simulink model "ECE411_ProjectTemplateSim2"  (R2021b)
settings: Solver=FixedStepDiscrete  StartTime=0.0  StopTime=10  FixedStep=Ts  RelTol=1e-3  EnableMultiTasking=on
PreLoadFcn:
  | ee_bldc_speed_control_data;
StopFcn:
  | ee_addSimlogTimeStamp(bdroot)
values from neighbouring files (symbols this model uses):
  Bm = 42e-3    (= 0.042)    [Wooter_parameters.m]
  Drive_Idc_limit = 200    [Wooter_parameters.m]
  eff_radius = r_wheel/G_ratio    (= 0.034375)    [Wooter_parameters.m]
  I_cmd_manual_step = 133    [Wooter_parameters.m]
  Ki_Idc_Regulator = 5.723    [Wooter_parameters.m]
  Ki_vel_Regulator = 5    [Wooter_parameters.m]
  Kp_Idc_Regulator = 0.286    [Wooter_parameters.m]
  Kp_vel_Regulator = 5    [Wooter_parameters.m]
  p = 4    [Wooter_parameters.m]
  RPM_max = 4259    [Wooter_parameters.m]
  tau_Te_filter = 1/(2*pi*10)    (= 0.0159154943092)    [Wooter_parameters.m]
  Tsc = 1e-4    (= 0.0001)    [Wooter_parameters.m]
  Vdc_max = 72    [Wooter_parameters.m]
  vel_0 = 0    [Wooter_parameters.m]
  vel_1 = 11.11    [Wooter_parameters.m]
  vel_2 = 13.889    [Wooter_parameters.m]
  vel_3 = 9.722    [Wooter_parameters.m]
libraries: nesl_utility x16, fl_lib x10, ee_lib x8, eeDiscretePi x2, eeGeneralControl x1
CloseFcn:
  | try,close(h1_ee_bldc_speed_control),end
  | clear h1_ee_bldc_speed_control
  | 
  | clear simlog_ee_bldc_speed_control
  | clear logsout_ee_bldc_speed_control
Description:
  | BLDC Speed Control
settings Model: Creator=The MathWorks, Inc.  LastModifiedBy=divad
settings SolverCC: AlgebraicLoopSolver=TrustRegion
settings DataIOCC: MaxDataPoints=210000  ReturnWorkspaceOutputs=off  SignalLoggingName=logsout_ee_bldc_speed_control
settings OptimizationCC: LifeSpan=inf
settings DebuggingCC: UnderspecifiedInitializationDetection=Classic  MergeDetectMultiDrivingBlocksExec=none  SFUnexpectedBacktrackingDiag=warning  SFNoUnconditionalDefaultTransitionDiag=warning  SFExecutionAtInitializationDiag=none  SFMachineParentedDataDiag=warning  ArithmeticOperatorsInVariantConditions=warning
settings SFSimCC: SimUseLocalCustomCode=off  CustomCodeUndefinedFunction=UseInterfaceOnly
settings RTWCC: RTWUseLocalCustomCode=off
settings CodeAppCC: StateflowObjectComments=on
settings GRTTargetCC: TargetLangStandard=C89/C90 (ANSI)
settings ConfigComp: CovMetricSettings=dw  CovSaveCumulativeToWorkspaceVar=on  CovSaveSingleToWorkspaceVar=on  CovExternalEMLEnable=off
settings SimscapeCC: SimscapeNormalizeSystem=off  SimscapeLogType=all  SimscapeLogSimulationStatistics=on  SimscapeLogName=simlog_ee_bldc_speed_control  SimscapeLogDataHistory=210000

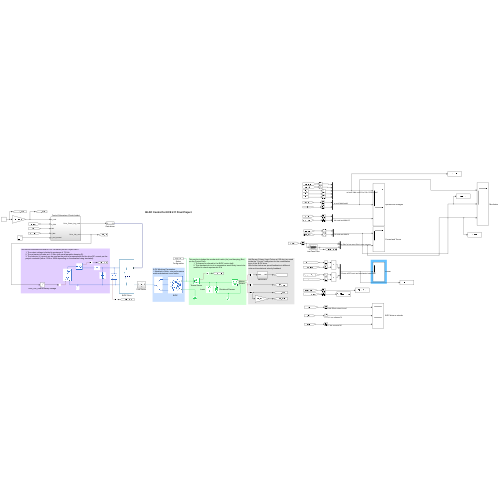
[thumbnail: Simulink's stored preview of the top-level diagram]
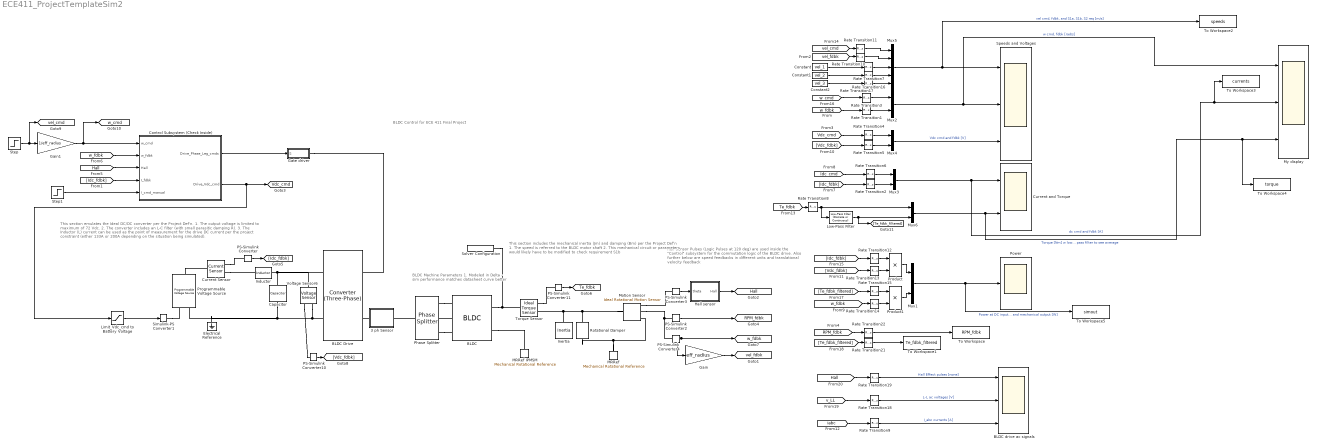
== system ECE411_ProjectTemplateSim2 ==
  note: Hall Sensor Pulses (Logic Pulses at 120 deg) are used inside the "Control" subsystem for the commutation logic of the BLDC drive.
      | Also further below are speed feedbacks in different units and translational velocity feedback
  note: This section emulates the Ideal DC/DC converter per the Project Def'n.
      | 1. The output voltage is limited to maximum of 72 Vdc.
      | 2. The converter includes an L-C filter (with small parasitic damping R).
      | 3. The Inductor (L) current can be used as the point of measurement for the drive DC current per the project constraint (either 133A or 200A depending on the situation being simulated).
  note: BLDC Control for ECE 411 Final Project
  note: This section includes the mechanical inertia (Jm) and damping (Bm) per the Project Def'n
      | 1. The speed is referred to the BLDC motor shaft
      | 2. This mechanical circuit or parameters would likely have to be modified to check requirement S1b
  note: BLDC Machine Parameters
      | 1. Modeled in Delta - sim performance matches datasheet curve better
  3 ph Sensor : Subsystem
  BLDC : ee_lib/Electromechanical/Permanent Magnet/BLDC  port_option=ee.enum.threePhasePort.expanded  winding_type=ee.enum.statorconnection.delta  rotor_param=ee.enum.pmsm.backemf.trapezoidbackemf  pm_flux_linkage=0.175 N*m/A  theta_constant=pi / (2*p) rad  emf_max=Vdc_max V  w_meas=RPM_max rpm  DphiDtheta_tab=[0, -.1528, -.1528, .1528, .1528, 0] Wb/rad  back_emf_tab=[0, -9.6, -9.6, 9.6, 9.6, 0] V  rotor_angle_tab=[0, 7.5, 22.5, 37.5, 52.5, 60] deg  nPolePairs=p  axes_param=ee.enum.rotorangle.qaxis  stator_param=ee.enum.statorparam.LsLmMs  machine_param=ee.enum.dqparameterization.constant  Ld=0.00022 H  Lq=0.00022 H  idVec=[-200, 0, 200] A  iqVec=[-200, 0, 200] A  LdMatrix=0.00022 * ones(3, 3) H  LqMatrix=0.00022 * ones(3, 3) H  L0=0.00016 H  Ls=Ls H  Lm=0 H  Ms=Ms H  Rs=Rs Ohm  zero_sequence=ee.enum.park.zerosequence.exclude  loss_param=ee.enum.ironloss.none  losses_oc=[0, 0, 0] W  losses_sc=[0, 0, 0] W  f_losses=60 Hz  Isc_losses=95 A  J=0 kg*m^2  lam=0 N*m/(rad/s)  i_d_specify=off  i_d_priority=None  i_d=0 A  i_d_nominal_specify=off  i_d_nominal_unit=A  i_d_nominal_value=1  i_q_specify=off  i_q_priority=None  i_q=0 A  i_q_nominal_specify=off  i_q_nominal_unit=A  i_q_nominal_value=1  torque_specify=off  torque_priority=None  torque=0 N*m  torque_nominal_specify=off  torque_nominal_unit=N*m  torque_nominal_value=1  angular_velocity_specify=off  angular_velocity_priority=High  angular_velocity=RPM_max*1e6 rpm  angular_velocity_nominal_specify=off  angular_velocity_nominal_unit=rpm  angular_velocity_nominal_value=1  angular_position_specify=off  angular_position_priority=High  angular_position=0 deg  angular_position_nominal_specify=off  angular_position_nominal_unit=deg  angular_position_nominal_value=1  alpha=3.93e-3 1/K  alpha_flux=-0.001 1/K  Tmeas=298.15 K  stator_thermal_mass=100 J/K  rotor_thermal_mass=200 J/K  Rm_percent_rotor=90  Rd_percent_rotor=30  temperatureA_specify=off  temperatureA_priority=High  temperatureA=25 degC  temperatureA_nominal_specify=off  temperatureA_nominal_unit=degC  temperatureA_nominal_value=1  temperatureB_specify=off  temperatureB_priority=High  temperatureB=25 degC  temperatureB_nominal_specify=off  temperatureB_nominal_unit=degC  temperatureB_nominal_value=1  temperatureC_specify=off  temperatureC_priority=High  temperatureC=25 degC  temperatureC_nominal_specify=off  temperatureC_nominal_unit=degC  temperatureC_nominal_value=1  temperatureR_specify=off  temperatureR_priority=High  temperatureR=25 degC  temperatureR_nominal_specify=off  temperatureR_nominal_unit=degC  temperatureR_nominal_value=1
      settings: SourceProductBaseCode=PS  InternalSimscapePortConfiguration="{\"Bottom\":[],\"Left\":[{\"id\":\"a\",\"label\":\"a\",\"type\":\"foundation.electrical.electrical\"},{\"id\":\"b\",\"label\":\"b\",\"type\":\"foundation.electrical.electrical\"},{\"id\":\"c\",\"label\":\"c\",\"type\":\"foundation.electrical.electrical\"}],\"Right\":[{\"id\":\"R\",\"label\":\"R\",\"type\":\"foundation.mechanical.rotational.rotational\"},{\"id\":\"C\",\"label\":\"C\",\"type\":\"foundation.mechanical.rotational.rotational\"}],\"Top\":[]}"
  BLDC Drive : ee_lib/Semiconductors & Converters/Converters/Converter (Three-Phase)  port_option=ee.enum.threePhasePort.composite  device_type=ee.enum.converters.switchingdevice.ideal  Vf=Vf_IGBT V  Ron=Ron_IGBT Ohm  Rds=0.001 Ohm  Goff=1e-5 1/Ohm  Vgt=1 V  Vgt_off=-1 V  Ih=1 A  Vth=0.5 V  diode_param=ee.enum.converters.protectiondiode.nodynamics  diode_Vf=Vf_Diode V  diode_Ron=Ron_Diode Ohm  diode_Goff=1e-5 1/Ohm  diode_C=50 nF  diode_iRM=-235 A  diode_iF=300 A  diode_idot=-50 A/us  diode_trr_param=ee.enum.converters.diodetrr.trr_factor  diode_trr_factor=3  diode_trr=15 us  diode_Qrr=1.5e+3 s*uA  snubber_type=ee.enum.converters.snubber.exclude  Cs=1e-7 F  Rs=0.1 Ohm
      settings: SourceProductBaseCode=PS
  BLDC drive ac signals : Scope  NumInputPorts=3
  Capacitor : fl_lib/Electrical/Electrical Elements/Capacitor  c=500e-3 F  r=1e-6 Ohm  g=0 1/Ohm  i_specify=off  i_priority=None  i=0 A  i_nominal_specify=off  i_nominal_unit=A  i_nominal_value=1  v_specify=on  v_priority=None  v=0 V  v_nominal_specify=off  v_nominal_unit=V  v_nominal_value=1  vc_specify=off  vc_priority=High  vc=0 V  vc_nominal_specify=off  vc_nominal_unit=V  vc_nominal_value=1
  Constant : Constant  Value=vel_1
  Constant1 : Constant  Value=vel_2
  Constant2 : Constant  Value=vel_3
  Control Subsystem (Check Inside) : Subsystem
  Current Sensor : fl_lib/Electrical/Electrical Sensors/Current Sensor
  Current and Torque : Scope  NumInputPorts=2
  Electrical Reference : fl_lib/Electrical/Electrical Elements/Electrical Reference
  Gain : Gain  Gain=eff_radius
  Gain1 : Gain  Gain=1/eff_radius
  Gate driver : Subsystem
  Hall sensor : Subsystem
  Inductor : ee_lib/Passive/Inductor  l=1e-3 H  L_tol=20  enable_L_tol=0  tol_distribution=1  nSigma=4  r=1e-3 Ohm  g=1e-9 1/Ohm  enable_operating_limits=0  operating_limit_action=2  max_working_current=1 A  power_rating=1 W  enable_faults=0  fault_action=1  lambdaPercent=50  k_faulted=0.9999  turnsShort=0  openCct=0  groundShort=0  groundShortG=0 1/Ohm  tau_fault=1e-3 s  enable_temporal_fault=0  t_fault=1 s  enable_behavioral_fault=0  max_permissible_voltage=100 V  n_fail_on_voltage=1  max_permissible_current=1 A  t_fail_on_current=1 s  i_L_specify=off  i_L_priority=High  i_L=0 A  i_L_nominal_specify=off  i_L_nominal_unit=A  i_L_nominal_value=1
  Inertia : fl_lib/Mechanical/Rotational Elements/Inertia  inertia=Jm kg*m^2  num_ports=foundation.enum.numPorts2.one  w_specify=on  w_priority=High  w=0 rpm  w_nominal_specify=off  w_nominal_unit=rad/s  w_nominal_value=1  t_specify=off  t_priority=High  t=0 N*m  t_nominal_specify=off  t_nominal_unit=N*m  t_nominal_value=1
  Limit_Vdc_cmd to Battery Voltage : Saturate  UpperLimit=Vdc_max  LowerLimit=0
  Low-Pass Filter : eeGeneralControl/Low-Pass Filter (Discrete or Continuous)  K=1  T=tau_Te_filter  B=inf  A=-inf  init_option=Inherited from block input  x0=0  Ts=-1
  MRRef : fl_lib/Mechanical/Rotational Elements/Mechanical Rotational Reference
  MRRef IPMSM : fl_lib/Mechanical/Rotational Elements/Mechanical Rotational Reference
  Motion Sensor : fl_lib/Mechanical/Mechanical Sensors/Ideal Rotational Motion Sensor  wrap_angle=simscape.enum.onoff.off  offset=0 deg
  Mux{1..4,6} (5 alike) : Mux  Inputs=2
  Mux5 : Mux  Inputs=5
  My display : Scope  NumInputPorts=3
  PS-Simulink Converter : nesl_utility/PS-Simulink Converter  PhysicalDomain=network_engine_domain  SubClassName=ps_output  LeftPortType=input  RightPortType=output  PseudoPeriodic=off  Frequencies=[]  Unit=A  AffineConversion=off
      settings: SourceProductBaseCode=PW,SS
  PS-Simulink Converter10 : nesl_utility/PS-Simulink Converter  PhysicalDomain=network_engine_domain  SubClassName=ps_output  LeftPortType=input  RightPortType=output  PseudoPeriodic=off  Frequencies=[]  Unit=V  AffineConversion=off
      settings: SourceProductBaseCode=PW,SS
  PS-Simulink Converter11 : nesl_utility/PS-Simulink Converter  PhysicalDomain=network_engine_domain  SubClassName=ps_output  LeftPortType=input  RightPortType=output  PseudoPeriodic=off  Frequencies=[]  Unit=N*m  AffineConversion=off
      settings: SourceProductBaseCode=PW,SS
  PS-Simulink Converter2 : nesl_utility/PS-Simulink Converter  PhysicalDomain=network_engine_domain  SubClassName=ps_output  LeftPortType=input  RightPortType=output  PseudoPeriodic=off  Frequencies=[]  Unit=rpm  AffineConversion=off
      settings: SourceProductBaseCode=PW,SS
  PS-Simulink Converter3 : nesl_utility/PS-Simulink Converter  PhysicalDomain=network_engine_domain  SubClassName=ps_output  LeftPortType=input  RightPortType=output  PseudoPeriodic=off  Frequencies=[]  Unit=rad  AffineConversion=off
      settings: SourceProductBaseCode=PW,SS
  PS-Simulink Converter4 : nesl_utility/PS-Simulink Converter  PhysicalDomain=network_engine_domain  SubClassName=ps_output  LeftPortType=input  RightPortType=output  PseudoPeriodic=off  Frequencies=[]  Unit=rad/s  AffineConversion=off
      settings: SourceProductBaseCode=PW,SS
  Phase Splitter : ee_lib/Connectors & References/Phase Splitter
      settings: SourceProductBaseCode=PS
  Power : Scope
  Product : Product
  Product1 : Product
  Programmable Voltage Source : ee_lib/Sources/Programmable Voltage Source  magnitude_type=ee.enum.timechanging.constant  ac_magnitude=0 V  magn_ramp=1 V/s  magn_step=1 V  magn_modu_magn=1 V  magn_modu_freq=1 Hz  magn_t1=1 s  magn_t2=2 s  frequency_type=ee.enum.timechanging.constant  ac_frequency=1 Hz  freq_ramp=1 Hz/s  freq_step=1 Hz  freq_modu_magn=1 Hz  freq_modu_freq=1 Hz  freq_t1=1 s  freq_t2=2 s  phase_type=ee.enum.timechanging.constant  ac_shift=0 deg  phase_ramp=1 deg/s  phase_step=1 deg  phase_modu_magn=1 deg  phase_modu_freq=1 Hz  phase_t1=1 s  phase_t2=2 s  dc_type=ee.enum.timechanging.external  dc_voltage=0 V  dc_ramp=1 V/s  dc_step=1 V  dc_modu_magn=1 V  dc_modu_freq=1 Hz  dc_t1=1 s  dc_t2=2 s  harmonic_option=0  harmonic_orders=[5, 7, 11, 13]  harmonic_ratios=[.1, .1, .1, .1]  harmonic_shifts=[0, 0, 0, 0] deg  harmonic_t1=-inf s  harmonic_t2=inf s  noise_mode=0  PSD=0 V^2/Hz  repeatability=1  auto_seed=0  user_seed=0  sample_time=1e-3 s  i_specify=off  i_priority=None  i=0 A  i_nominal_specify=off  i_nominal_unit=A  i_nominal_value=1  v_specify=on  v_priority=None  v=0 V  v_nominal_specify=off  v_nominal_unit=V  v_nominal_value=1
      settings: SourceProductBaseCode=PS  InternalSimscapePortConfiguration="{\"Bottom\":[],\"Left\":[{\"id\":\"p\",\"label\":\"+\",\"type\":\"foundation.electrical.electrical\"}],\"Right\":[{\"id\":\"ext_dc\",\"label\":\"DC\",\"type\":\"input\"},{\"id\":\"n\",\"label\":\"-\",\"type\":\"foundation.electrical.electrical\"}],\"Top\":[]}"
  Rate Transition{1,3,7,10..17} (11 alike) : RateTransition
  Rate Transition{2,4..6,8..9,18..19,21..22} (10 alike) : RateTransition  OutPortSampleTime=1e-4
  Rotational Damper : fl_lib/Mechanical/Rotational Elements/Rotational Damper  D=Bm N*m/(rad/s)  w_specify=off  w_priority=None  w=0 rad/s  w_nominal_specify=off  w_nominal_unit=rad/s  w_nominal_value=1  t_specify=off  t_priority=None  t=0 N*m  t_nominal_specify=off  t_nominal_unit=N*m  t_nominal_value=1
  Simulink-PS Converter1 : nesl_utility/Simulink-PS Converter  PhysicalDomain=network_engine_domain  SubClassName=ps_input  LeftPortType=input  RightPortType=output  PseudoPeriodic=off  Frequencies=[]  NoiseDistribution=none  NoiseParameters=[]  Unit=V  AffineConversion=off  FilteringAndDerivatives=zero  SimscapeFilterOrder=1  InputFilterTimeConstant=0.001  UdotUserProvided=1
      settings: SourceProductBaseCode=PW,SS
  Solver Configuration : nesl_utility/Solver Configuration  PhysicalDomain=network_engine_domain  SubClassName=solver  LeftPortType=input  RightPortType=generic  Tones=[]  Harmonics=[]  SimulateNoise=off  Profile=off  UseLocalSampling=off  EnableSwitchedLinearOptims=on  FrequencyDomain=off  UseCCode=off  RelTol=0.001  AbsTol=1e-06  MinStep=1e-09  ToWorkspace=off  RevertToSquareIcSolve=off  NumHomotopyIterations=100  PhasorMode=off  PhasorModeNumHarmonics=1  DoDC=off  ResidualTolerance=1e-09  UseLocalSolver=on  LocalSolverChoice=NE_TRAPEZOIDAL_ADVANCER  LocalSolverSampleTime=1e-5  DoFixedCost=on  MaxNonlinIter=3  MaxModeIter=2  ComputeImpulses=off  ImpulseIterations=2  LinearAlgebra=auto  EquationFormulation=NE_TIME_EF  DelaysMemoryBudget=1024  AutomaticFiltering=on  FilteringTimeConstant=0.001  PartitionStorageMethod=AS_NEEDED  PartitionMemoryBudget=1024  PartitionMethod=ROBUST
      settings: SourceProductBaseCode=PW,SS
  Speeds and Voltages : Scope  NumInputPorts=3
  Step : Step  Before=vel_0  After=vel_1  SampleTime=0
  Step1 : Step  Time=0.5  After=I_cmd_manual_step  SampleTime=0
  To Workspace : ToWorkspace  VariableName=RPM_fdbk  SampleTime=-1
  To Workspace1 : ToWorkspace  VariableName=Te_fdbk_filtered  SampleTime=-1
  To Workspace2 : ToWorkspace  VariableName=speeds  SampleTime=-1
  To Workspace3 : ToWorkspace  VariableName=currents  SampleTime=-1
  To Workspace4 : ToWorkspace  VariableName=torque  SampleTime=-1
  To Workspace5 : ToWorkspace  VariableName=simout  SampleTime=-1
  Torque Sensor : fl_lib/Mechanical/Mechanical Sensors/Ideal Torque Sensor
  Voltage Sensor6 : fl_lib/Electrical/Electrical Sensors/Voltage Sensor
  tag scope: Hall=global, RPM_fdbk=global, Te_fdbk=global, Vdc_cmd=global, vel_cmd=global, vel_fdbk=global, w_cmd=global, w_fdbk=global
  wires:
  Control Subsystem (Check Inside)/1(Drive_Phase_Leg_cmds) -> Gate driver/1(S)
  [w_fdbk] -> Control Subsystem (Check Inside)/2(w_fdbk)
  [Hall] -> Control Subsystem (Check Inside)/3(Hall)
  [Idc_fdbk] -> Control Subsystem (Check Inside)/4(I_fdbk)
  PS-Simulink Converter/1 -> [Idc_fdbk]
  Control Subsystem (Check Inside)/2(Drive_Vdc_cmd) -> Limit_Vdc_cmd to Battery Voltage/1, [Vdc_cmd]
  Hall sensor/1(Hall) -> [Hall]
  PS-Simulink Converter3/1 -> Hall sensor/1(theta)
  PS-Simulink Converter2/1 -> [RPM_fdbk]
  [w_cmd] -> Rate Transition3/1
  Rate Transition1/1 -> Mux2/2
  [w_fdbk] -> Rate Transition1/1
  Mux3/1 -> To Workspace3/1, My display/2, Current and Torque/1  "dc cmd and fdbk [A]"
  [Idc_fdbk] -> Rate Transition2/1
  [Idc_cmd] -> Rate Transition6/1
  Rate Transition4/1 -> Mux4/1
  Rate Transition6/1 -> Mux3/1
  [Vdc_cmd] -> Rate Transition4/1
  Rate Transition2/1 -> Mux3/2
  PS-Simulink Converter11/1 -> [Te_fdbk]
  Product/1 -> Mux1/1
  Mux1/1 -> To Workspace5/1, Power/1  "Power at DC input and mechanical output [W]"
  [w_fdbk] -> Rate Transition14/1
  [Te_fdbk_filtered] -> Rate Transition15/1
  Product1/1 -> Mux1/2
  PS-Simulink Converter10/1 -> [Vdc_fdbk]
  [Vdc_fdbk] -> Rate Transition5/1
  Rate Transition5/1 -> Mux4/2
  Mux4/1 -> Speeds and Voltages/3  "Vdc cmd and fdbk [V]"
  [Vdc_fdbk] -> Rate Transition13/1
  Mux5/1 -> To Workspace2/1, Speeds and Voltages/1  "vel cmd, fdbk, and S1a, S1b, S2 req [m/s]"
  [Te_fdbk] -> Rate Transition8/1
  PS-Simulink Converter4/1 -> Gain/1, [w_fdbk]
  [iabc] -> Rate Transition9/1
  Step1/1 -> Control Subsystem (Check Inside)/5(I_cmd_manual)
  Limit_Vdc_cmd to Battery Voltage/1 -> Simulink-PS Converter1/1
  Step/1 -> [vel_cmd], Gain1/1
  Gain/1 -> [vel_fdbk]
  Gain1/1 -> [w_cmd], Control Subsystem (Check Inside)/1(w_cmd)
  Rate Transition3/1 -> Mux2/1
  [vel_fdbk] -> Rate Transition10/1
  Constant/1 -> Rate Transition7/1
  Rate Transition7/1 -> Mux5/3
  Rate Transition10/1 -> Mux5/2
  [vel_cmd] -> Rate Transition11/1
  Rate Transition11/1 -> Mux5/1
  Mux2/1 -> My display/1, Speeds and Voltages/2  "w cmd, fdbk [rad/s]"
  Low-Pass Filter/1 -> [Te_fdbk_filtered], Mux6/2
  Mux6/1 -> To Workspace4/1, My display/3, Current and Torque/2  "Torque [Nm] w low pass filter to see average"
  Rate Transition13/1 -> Product/2
  [Idc_fdbk] -> Rate Transition12/1
  Rate Transition12/1 -> Product/1
  Rate Transition14/1 -> Product1/2
  Rate Transition15/1 -> Product1/1
  Constant1/1 -> Rate Transition16/1
  Rate Transition16/1 -> Mux5/4
  Constant2/1 -> Rate Transition17/1
  Rate Transition17/1 -> Mux5/5
  [RPM_fdbk] -> Rate Transition22/1
  [Te_fdbk_filtered] -> Rate Transition21/1
  [v_LL] -> Rate Transition18/1
  [Hall] -> Rate Transition19/1
  Rate Transition19/1 -> BLDC drive ac signals/1  "Hall Effect pulses [none]"
  Rate Transition18/1 -> BLDC drive ac signals/2  "L-L ac voltages [V]"
  Rate Transition9/1 -> BLDC drive ac signals/3  "I_abc currents [A]"
  Rate Transition8/1 -> Mux6/1, Low-Pass Filter/1
  Rate Transition21/1 -> To Workspace1/1
  Rate Transition22/1 -> To Workspace/1
  connections:
  Gate driver/RConn1 -- BLDC Drive/LConn1
  BLDC/RConn2 -- MRRef IPMSM/LConn1
  BLDC/RConn1 -- Solver Configuration/RConn1 -- Torque Sensor/LConn1
  Voltage Sensor6/RConn2 -- Electrical Reference/LConn1 -- Programmable Voltage Source/RConn2 -- Capacitor/RConn1 -- BLDC Drive/RConn2
  Programmable Voltage Source/LConn1 -- Current Sensor/LConn1
  Current Sensor/RConn1 -- PS-Simulink Converter/LConn1
  BLDC/LConn2 -- Phase Splitter/RConn2
  Simulink-PS Converter1/RConn1 -- Programmable Voltage Source/RConn1
  Capacitor/LConn1 -- Inductor/RConn1 -- Voltage Sensor6/LConn1 -- BLDC Drive/RConn1
  Motion Sensor/RConn3 -- PS-Simulink Converter3/LConn1
  Motion Sensor/RConn2 -- PS-Simulink Converter4/LConn1 -- PS-Simulink Converter2/LConn1
  MRRef/LConn1 -- Rotational Damper/RConn1 -- Motion Sensor/RConn1
  Motion Sensor/LConn1 -- Rotational Damper/LConn1 -- Inertia/LConn1 -- Torque Sensor/RConn1
  Phase Splitter/RConn3 -- BLDC/LConn3
  Phase Splitter/RConn1 -- BLDC/LConn1
  Voltage Sensor6/RConn1 -- PS-Simulink Converter10/LConn1
  Torque Sensor/RConn2 -- PS-Simulink Converter11/LConn1
  Current Sensor/RConn2 -- Inductor/LConn1
  3 ph Sensor/LConn1 -- BLDC Drive/LConn2
  Phase Splitter/LConn1 -- 3 ph Sensor/RConn1

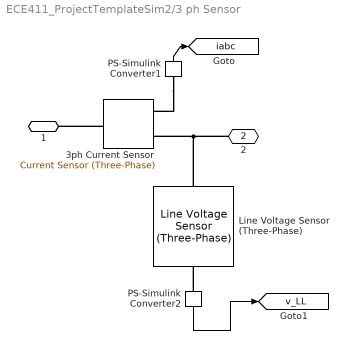
== system ECE411_ProjectTemplateSim2/3 ph Sensor ==
  3ph Current Sensor : ee_lib/Sensors & Transducers/Current Sensor (Three-Phase)
  Line Voltage Sensor (Three-Phase) : ee_lib/Sensors & Transducers/Line Voltage Sensor (Three-Phase)
      settings: SourceProductBaseCode=PS
  PS-Simulink Converter1 : nesl_utility/PS-Simulink Converter  PhysicalDomain=network_engine_domain  SubClassName=ps_output  LeftPortType=input  RightPortType=output  PseudoPeriodic=off  Frequencies=[]  Unit=A  AffineConversion=off
      settings: SourceProductBaseCode=PW,SS
  PS-Simulink Converter2 : nesl_utility/PS-Simulink Converter  PhysicalDomain=network_engine_domain  SubClassName=ps_output  LeftPortType=input  RightPortType=output  PseudoPeriodic=off  Frequencies=[]  Unit=V  AffineConversion=off
      settings: SourceProductBaseCode=PW,SS
  1 : PMIOPort  Side=Left
  2 : PMIOPort  Port=2  Side=Right
  tag scope: iabc=global, v_LL=global
  wires:
  PS-Simulink Converter1/1 -> [iabc]
  PS-Simulink Converter2/1 -> [v_LL]
  connections:
  PS-Simulink Converter1/LConn1 -- 3ph Current Sensor/RConn1
  3ph Current Sensor/LConn1 -- 1/RConn1
  2/RConn1 -- Line Voltage Sensor (Three-Phase)/LConn1 -- 3ph Current Sensor/RConn2
  PS-Simulink Converter2/LConn1 -- Line Voltage Sensor (Three-Phase)/RConn1

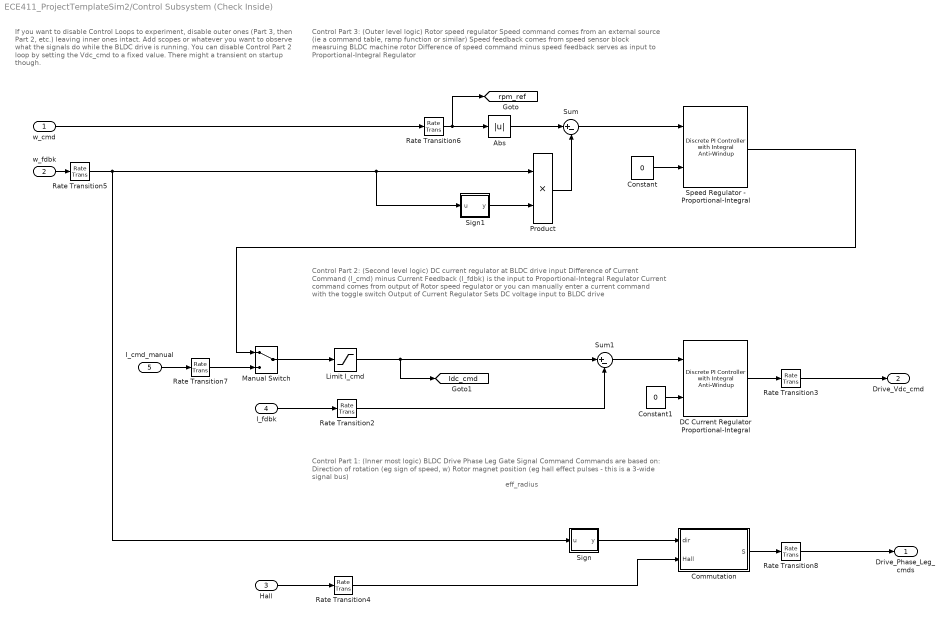
== system ECE411_ProjectTemplateSim2/Control Subsystem (Check Inside) ==
  note: If you want to disable Control Loops to experiment, disable outer ones (Part 3, then Part 2, etc.) leaving inner ones intact.  Add scopes or whatever you want to observe what the signals do while the BLDC drive is running.
      | You can disable Control Part 2 loop by setting the Vdc_cmd to a fixed value.  There might a transient on startup though.
  note: Control Part 1: (Inner most logic) BLDC Drive Phase Leg Gate Signal Command
      | Commands are based on:
      | Direction of rotation (eg sign of speed, w)
      | Rotor magnet position (eg hall effect pulses - this is a 3-wide signal bus)
  note: eff_radius
  note: Control Part 2: (Second level logic) DC current regulator at BLDC drive input
      | Difference of Current Command (I_cmd) minus Current Feedback (I_fdbk) is the input to Proportional-Integral Regulator
      | Current command comes from output of Rotor speed regulator or you can manually enter a current command with the toggle switch
      | Output of Current Regulator Sets DC voltage input to BLDC drive
  note: Control Part 3: (Outer level logic) Rotor speed regulator
      | Speed command comes from an external source (ie a command table, ramp function or similar)
      | Speed feedback comes from speed sensor block measruing BLDC machine rotor
      | Difference of speed command minus speed feedback serves as input to Proportional-Integral Regulator
  w_cmd : Inport
  w_fdbk : Inport  Port=2
  Hall : Inport  Port=3
  I_fdbk : Inport  Port=4
  I_cmd_manual : Inport  Port=5
  Abs : Abs
  Commutation : Subsystem
  Constant : Constant  Value=0  SampleTime=Tsc
  Constant1 : Constant  Value=0  SampleTime=Tsc
  DC Current Regulator Proportional-Integral : eeDiscretePi/Discrete PI Controller with Integral Anti-Windup  Kp=Kp_Idc_Regulator  Ki=Ki_Idc_Regulator  x0=0  B=Vdc_max  A=0  Ts=Tsc
      settings: SourceProductBaseCode=PS
  Limit I_cmd : Saturate  UpperLimit=Drive_Idc_limit  LowerLimit=0
  Manual Switch : ManualSwitch
  Product : Product
  Rate Transition{2..3,6..7} (4 alike) : RateTransition
  Rate Transition4 : RateTransition  OutPortSampleTime=Tsc
  Rate Transition5 : RateTransition  OutPortSampleTime=Tsc
  Rate Transition8 : RateTransition  OutPortSampleTime=Ts
  Sign : Subsystem
  Sign1 : Subsystem
  Speed Regulator - Proportional-Integral : eeDiscretePi/Discrete PI Controller with Integral Anti-Windup  Kp=Kp_vel_Regulator  Ki=Ki_vel_Regulator  x0=0  B=Drive_Idc_limit  A=0  Ts=Tsc
      settings: SourceProductBaseCode=PS
  Sum : Sum  Inputs=|+-
  Sum1 : Sum  Inputs=|+-
  Drive_Phase_Leg_cmds : Outport  VectorParamsAs1DForOutWhenUnconnected=off
  Drive_Vdc_cmd : Outport  Port=2  VectorParamsAs1DForOutWhenUnconnected=off
  tag scope: Idc_cmd=global, rpm_ref=global
  wires:
  Hall/1 -> Rate Transition4/1
  w_cmd/1 -> Rate Transition6/1
  Rate Transition6/1 -> Abs/1, [rpm_ref]
  Sum/1 -> Speed Regulator - Proportional-Integral/1
  Constant/1 -> Speed Regulator - Proportional-Integral/2
  Rate Transition8/1 -> Drive_Phase_Leg_cmds/1
  Rate Transition4/1 -> Commutation/2(Hall)
  I_fdbk/1 -> Rate Transition2/1
  Rate Transition2/1 -> Sum1/2
  Abs/1 -> Sum/1
  Product/1 -> Sum/2
  Rate Transition5/1 -> Sign1/1(u), Product/1, Sign/1(u)
  Sign/1(y) -> Commutation/1(dir)
  Commutation/1(S) -> Rate Transition8/1
  Manual Switch/1 -> Limit I_cmd/1
  w_fdbk/1 -> Rate Transition5/1
  Sum1/1 -> DC Current Regulator Proportional-Integral/1
  Constant1/1 -> DC Current Regulator Proportional-Integral/2
  Rate Transition3/1 -> Drive_Vdc_cmd/1
  DC Current Regulator Proportional-Integral/1 -> Rate Transition3/1
  Speed Regulator - Proportional-Integral/1 -> Manual Switch/1
  I_cmd_manual/1 -> Rate Transition7/1
  Rate Transition7/1 -> Manual Switch/2
  Limit I_cmd/1 -> [Idc_cmd], Sum1/1
  Sign1/1(y) -> Product/2

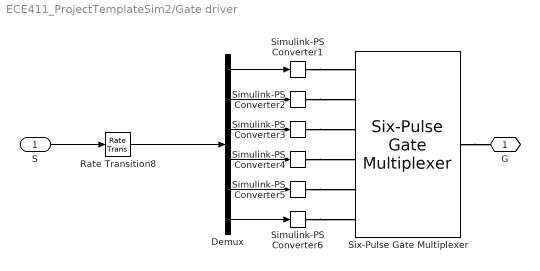
== system ECE411_ProjectTemplateSim2/Gate driver ==
  S : Inport
  Demux : Demux  Outputs=6
  Rate Transition8 : RateTransition
  Simulink-PS Converter{1..6} (6 alike) : nesl_utility/Simulink-PS Converter  PhysicalDomain=network_engine_domain  SubClassName=ps_input  LeftPortType=input  RightPortType=output  PseudoPeriodic=off  Frequencies=[]  NoiseDistribution=none  NoiseParameters=[]  Unit=1  AffineConversion=off  FilteringAndDerivatives=zero  SimscapeFilterOrder=1  InputFilterTimeConstant=0.001  UdotUserProvided=1
      settings: SourceProductBaseCode=PW,SS
  Six-Pulse Gate Multiplexer : ee_lib/Semiconductors & Converters/Converters/Six-Pulse Gate Multiplexer  port_option=ee.enum.controlport.ps
      settings: SourceProductBaseCode=PS
  G : PMIOPort  Side=Right
  wires:
  Demux/1 -> Simulink-PS Converter1/1
  Demux/4 -> Simulink-PS Converter4/1
  Demux/2 -> Simulink-PS Converter2/1
  Demux/3 -> Simulink-PS Converter3/1
  Demux/5 -> Simulink-PS Converter5/1
  Demux/6 -> Simulink-PS Converter6/1
  S/1 -> Rate Transition8/1
  Rate Transition8/1 -> Demux/1
  connections:
  Six-Pulse Gate Multiplexer/RConn1 -- G/RConn1
  Simulink-PS Converter1/RConn1 -- Six-Pulse Gate Multiplexer/LConn1
  Simulink-PS Converter3/RConn1 -- Six-Pulse Gate Multiplexer/LConn3
  Simulink-PS Converter5/RConn1 -- Six-Pulse Gate Multiplexer/LConn5
  Simulink-PS Converter6/RConn1 -- Six-Pulse Gate Multiplexer/LConn6
  Simulink-PS Converter4/RConn1 -- Six-Pulse Gate Multiplexer/LConn4
  Simulink-PS Converter2/RConn1 -- Six-Pulse Gate Multiplexer/LConn2

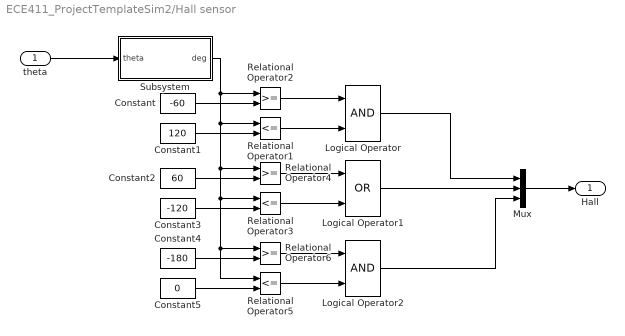
== system ECE411_ProjectTemplateSim2/Hall sensor ==
  theta : Inport
  Constant : Constant  Value=-60
  Constant1 : Constant  Value=120
  Constant2 : Constant  Value=60
  Constant3 : Constant  Value=-120
  Constant4 : Constant  Value=-180
  Constant5 : Constant  Value=0
  Logical Operator : Logic  AllPortsSameDT=off  OutDataTypeStr=boolean
  Logical Operator1 : Logic  Operator=OR  AllPortsSameDT=off  OutDataTypeStr=boolean
  Logical Operator2 : Logic  AllPortsSameDT=off  OutDataTypeStr=boolean
  Mux : Mux  Inputs=3
  Relational Operator1 : RelationalOperator  Operator=<=  RndMeth=Nearest  InputSameDT=on
  Relational Operator2 : RelationalOperator  RndMeth=Nearest  InputSameDT=on
  Relational Operator3 : RelationalOperator  Operator=<=  RndMeth=Nearest  InputSameDT=on
  Relational Operator4 : RelationalOperator  RndMeth=Nearest  InputSameDT=on
  Relational Operator5 : RelationalOperator  Operator=<=  RndMeth=Nearest  InputSameDT=on
  Relational Operator6 : RelationalOperator  RndMeth=Nearest  InputSameDT=on
  Subsystem : Subsystem
  Hall : Outport  VectorParamsAs1DForOutWhenUnconnected=off
  wires:
  Constant3/1 -> Relational Operator3/2
  Logical Operator2/1 -> Mux/3
  Logical Operator1/1 -> Mux/2
  Logical Operator/1 -> Mux/1
  Relational Operator5/1 -> Logical Operator2/2
  Relational Operator6/1 -> Logical Operator2/1
  Constant4/1 -> Relational Operator6/2
  Constant5/1 -> Relational Operator5/2
  Relational Operator3/1 -> Logical Operator1/2
  Mux/1 -> Hall/1
  Relational Operator2/1 -> Logical Operator/1
  Relational Operator1/1 -> Logical Operator/2
  Subsystem/1(deg) -> Relational Operator4/1, Relational Operator3/1, Relational Operator5/1, Relational Operator6/1, Relational Operator1/1, Relational Operator2/1
  Constant/1 -> Relational Operator2/2
  Relational Operator4/1 -> Logical Operator1/1
  Constant1/1 -> Relational Operator1/2
  Constant2/1 -> Relational Operator4/2
  theta/1 -> Subsystem/1(theta)

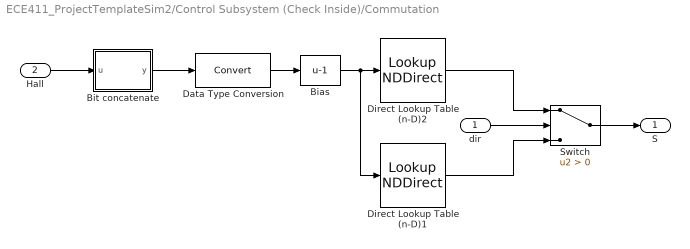
== system ECE411_ProjectTemplateSim2/Control Subsystem (Check Inside)/Commutation ==
  dir : Inport
  Hall : Inport  Port=2
  Bias : Bias  Bias=-1
  Bit concatenate : Subsystem
  Data Type Conversion : DataTypeConversion
  Direct Lookup Table (n-D)1 : LookupNDDirect  InputsSelectThisObjectFromTable=Vector  Table=[0 1 1 0 0 0;0 0 0 1 1 0;1 0 0 0 1 0;0 1 0 0 0 1;0 0 0 1 0 1;1 0 1 0 0 0]
  Direct Lookup Table (n-D)2 : LookupNDDirect  InputsSelectThisObjectFromTable=Vector  Table=[0 0 0 1 1 0;0 1 1 0 0 0;0 1 0 0 0 1;1 0 0 0 1 0;1 0 1 0 0 0;0 0 0 1 0 1]
  Switch : Switch  Criteria=u2 > Threshold
  S : Outport  VectorParamsAs1DForOutWhenUnconnected=off
  wires:
  Hall/1 -> Bit concatenate/1(u)
  Bit concatenate/1(y) -> Data Type Conversion/1
  Data Type Conversion/1 -> Bias/1
  Bias/1 -> Direct Lookup Table (n-D)1/1, Direct Lookup Table (n-D)2/1
  Switch/1 -> S/1
  dir/1 -> Switch/2
  Direct Lookup Table (n-D)2/1 -> Switch/1
  Direct Lookup Table (n-D)1/1 -> Switch/3

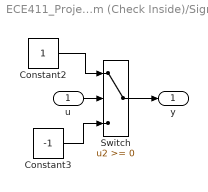
== system ECE411_ProjectTemplateSim2/Control Subsystem (Check Inside)/Sign ==
  u : Inport
  Constant2 : Constant
  Constant3 : Constant  Value=-1
  Switch : Switch
  y : Outport
  wires:
  Constant3/1 -> Switch/3
  Constant2/1 -> Switch/1
  u/1 -> Switch/2
  Switch/1 -> y/1

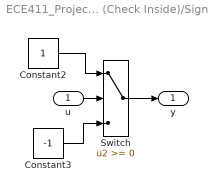
== system ECE411_ProjectTemplateSim2/Control Subsystem (Check Inside)/Sign1 ==
  u : Inport
  Constant2 : Constant
  Constant3 : Constant  Value=-1
  Switch : Switch
  y : Outport
  wires:
  Constant3/1 -> Switch/3
  Constant2/1 -> Switch/1
  u/1 -> Switch/2
  Switch/1 -> y/1

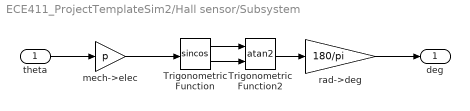
== system ECE411_ProjectTemplateSim2/Hall sensor/Subsystem ==
  theta : Inport
  Trigonometric Function : Trigonometry  Operator=sincos
  Trigonometric Function2 : Trigonometry  Operator=atan2
  mech->elec : Gain  Gain=p
  rad->deg : Gain  Gain=180/pi  SaturateOnIntegerOverflow=on  OutDataTypeStr=Inherit: Same as input  ParamDataTypeStr=Inherit: Same as input
  deg : Outport  VectorParamsAs1DForOutWhenUnconnected=off
  wires:
  Trigonometric Function2/1 -> rad->deg/1
  Trigonometric Function/1 -> Trigonometric Function2/1
  theta/1 -> mech->elec/1
  rad->deg/1 -> deg/1
  Trigonometric Function/2 -> Trigonometric Function2/2
  mech->elec/1 -> Trigonometric Function/1

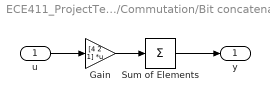
== system ECE411_ProjectTemplateSim2/Control Subsystem (Check Inside)/Commutation/Bit concatenate ==
  u : Inport
  Gain : Gain  Gain=[4 2 1]  Multiplication=Matrix(K*u)
  Sum of Elements : Sum  Inputs=+
  y : Outport  VectorParamsAs1DForOutWhenUnconnected=off
  wires:
  u/1 -> Gain/1
  Gain/1 -> Sum of Elements/1
  Sum of Elements/1 -> y/1
